simulink model "SimuEscalonContinuo"  (R2020a)
settings: Solver=VariableStepAuto  StartTime=0.0  StopTime=10  RelTol=1e-3
undefined symbols (not defined in the file): kd1, kd2, ki, kp, mu, tm
settings Model: Creator=Alexander  LastModifiedBy=AsusPC
settings DataIOCC: ReturnWorkspaceOutputs=off
settings DebuggingCC: ArithmeticOperatorsInVariantConditions=warning
settings SFSimCC: SimUseLocalCustomCode=off  CustomCodeUndefinedFunction=UseInterfaceOnly
settings RTWCC: RTWUseLocalCustomCode=off

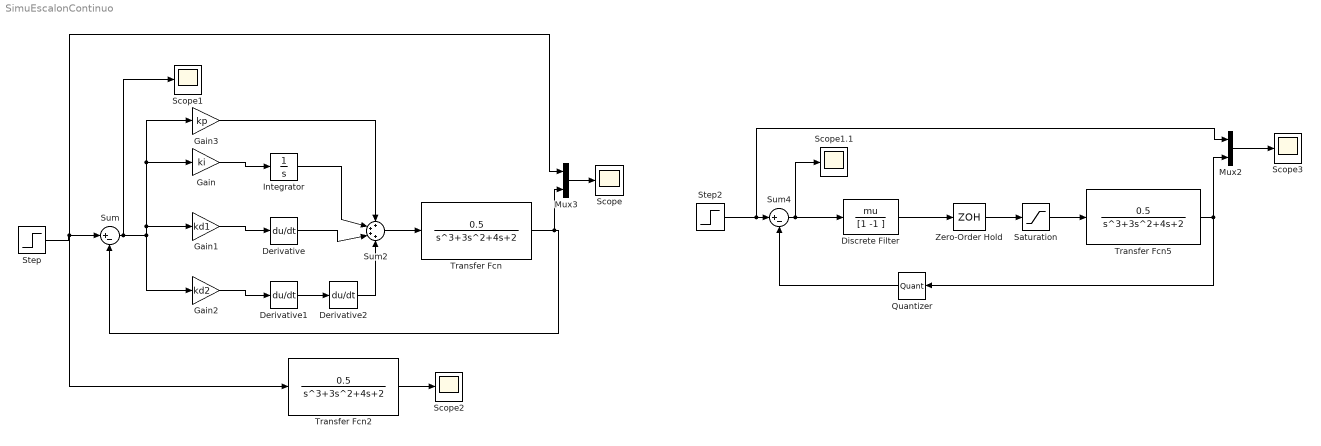
== system SimuEscalonContinuo ==
  Derivative : Derivative
  Derivative1 : Derivative
  Derivative2 : Derivative
  Discrete Filter : DiscreteFilter  Numerator=mu  Denominator=[1 -1 ]  SampleTime=tm
  Gain : Gain  Gain=ki
  Gain1 : Gain  Gain=kd1
  Gain2 : Gain  Gain=kd2
  Gain3 : Gain  Gain=kp
  Integrator : Integrator
  Mux2 : Mux  Inputs=2
  Mux3 : Mux  Inputs=2
  Quantizer : Quantizer  QuantizationInterval=3.3/1024
  Saturation : Saturate  UpperLimit=20  LowerLimit=-20
  Scope{,1..3} (4 alike) : Scope
  Scope1.1 : Scope
  Step : Step  Time=0  SampleTime=0
  Step2 : Step  Time=0  SampleTime=0
  Sum : Sum  Inputs=|+-
  Sum2 : Sum  Inputs=++++
  Sum4 : Sum  Inputs=|+-
  Transfer Fcn : TransferFcn  Numerator=[0.5]  Denominator=[1 3 4 2]
  Transfer Fcn2 : TransferFcn  Numerator=[0.5]  Denominator=[1 3 4 2]
  Transfer Fcn5 : TransferFcn  Numerator=[0.5]  Denominator=[1 3 4 2]
  Zero-Order Hold : ZeroOrderHold  SampleTime=tm
  wires:
  Sum4/1 -> Scope1.1/1, Discrete Filter/1
  Discrete Filter/1 -> Zero-Order Hold/1
  Transfer Fcn5/1 -> Quantizer/1, Mux2/2
  Mux2/1 -> Scope3/1
  Step2/1 -> Mux2/1, Sum4/1
  Zero-Order Hold/1 -> Saturation/1
  Quantizer/1 -> Sum4/2
  Saturation/1 -> Transfer Fcn5/1
  Transfer Fcn2/1 -> Scope2/1
  Transfer Fcn/1 -> Mux3/2, Sum/2
  Sum2/1 -> Transfer Fcn/1
  Step/1 -> Mux3/1, Sum/1, Transfer Fcn2/1
  Sum/1 -> Gain2/1, Gain1/1, Gain/1, Gain3/1, Scope1/1
  Gain/1 -> Integrator/1
  Gain1/1 -> Derivative/1
  Gain2/1 -> Derivative1/1
  Derivative1/1 -> Derivative2/1
  Derivative2/1 -> Sum2/4
  Derivative/1 -> Sum2/3
  Integrator/1 -> Sum2/2
  Gain3/1 -> Sum2/1
  Mux3/1 -> Scope/1
